simulink model "Rectiafier"  (R2024b)
settings: Solver=VariableStepAuto  StartTime=0.0  StopTime=0.1  RelTol=1e-3
libraries: spsThyristorLib x4, spsVoltageMeasurementLib x3, spsACVoltageSourceLib x1, dspswit3 x1, spsSeriesRLCBranchLib x1, spsUniversalBridgeLib x1, sps_lib x1
settings Model: Creator=Ahmad  LastModifiedBy=Ahmad

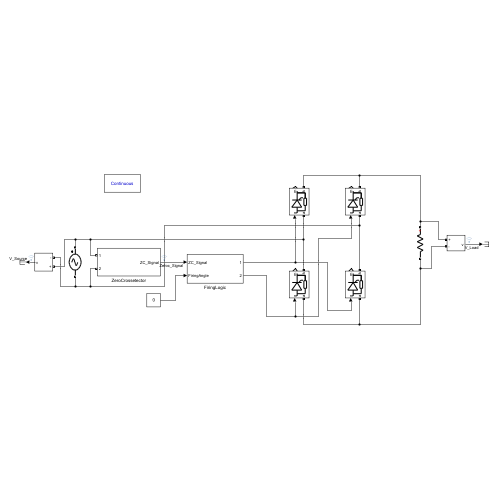
[thumbnail: Simulink's stored preview of the top-level diagram]
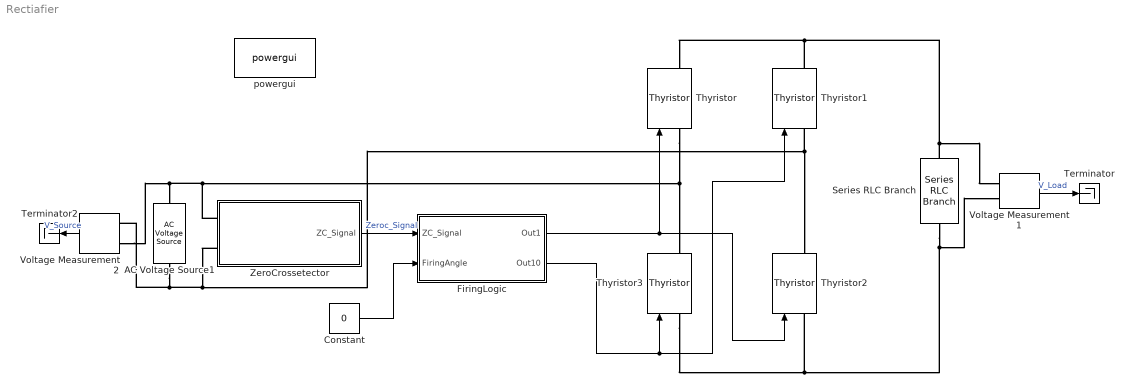
== system Rectiafier ==
  AC Voltage Source1 : spsACVoltageSourceLib/AC Voltage Source  Amplitude=sqrt(2)*220  Phase=0  Frequency=50  SampleTime=0  Measurements=None  BusType=swing  Pref=10e3  Qref=0  Qmin=-inf  Qmax=+inf
  Constant : Constant  Value=0
  FiringLogic : Subsystem
  Series RLC Branch : spsSeriesRLCBranchLib/Series RLC Branch  LConnTagsString=__new0  RConnTagsString=__new0  BranchType=R  Resistance=1  Inductance=1e-3  SetiL0=off  InitialCurrent=0  Capacitance=1e-6  Setx0=off  InitialVoltage=0  Measurements=None
  Terminator : Terminator
  Terminator2 : Terminator
  Thyristor{,1..3} (4 alike) : spsThyristorLib/Thyristor  Ron=0.001  Lon=0  Vf=0.8  IC=0  Rs=500  Cs=250e-9  Measurements=on
  Voltage Measurement1 : spsVoltageMeasurementLib/Voltage Measurement  PhasorSimulation=off  OutputType=Complex  PSBequivalent=0
  Voltage Measurement2 : spsVoltageMeasurementLib/Voltage Measurement  PhasorSimulation=off  OutputType=Complex  PSBequivalent=0
  ZeroCrossetector : Subsystem
  powergui : sps_lib/powergui  Priority=1  SimulationMode=Continuous  SampleTime=50e-6  frequency=60  Iterations=50  frequencyindice=0  Pbase=100e6  ErrMax=1e-4  UnitsV=kV  UnitsW=MW  buscounter=0  FunctionMessages=off  echomessages=off  EnableUseOfTLC=off  CurrentSourceSwitches=off  DisableSnubberDevices=off  DisableRonSwitches=off  DisableVfSwitches=off  DisplayEquations=off  AutomaticDiscreteSolvers=off  SolverType=Tustin/Backward Euler (TBE)  Interpol=off  ExternalGateDelay=off  methode=off  Ts=100  x0status=blocks  SPID=on  SwTol=0  HookPort=off  NonlinearTolerance=1e-4  nMaxIteration=100  ContinueOnMaxIteration=off  RestoreLinks=warning  ResistiveCurrentMeasurement=off  Frange=[0:2:500]  Ylog=off  Xlog=on  ShowGrid=off  save=off  variable=ZData  structure=0  ZoomFFT=off  StartTime=0.0  cycles=1  DisplayStyle=1  fundamental=60  FreqAxis=off  MaxFrequency=1000  frequencyindicesteady=1  RmsSteady=1  display=off
  wires:
  Voltage Measurement1/1 -> Terminator/1  "V_Load"
  Voltage Measurement2/1 -> Terminator2/1  "V_Source"
  ZeroCrossetector/1(ZC_Signal) -> FiringLogic/1(ZC_Signal)  "Zeroc_Signal"
  Constant/1 -> FiringLogic/2(FiringAngle)
  FiringLogic/1(Out1) -> Thyristor2/1, Thyristor/1
  FiringLogic/2(Out10) -> Thyristor1/1, Thyristor3/1
  connections:
  Voltage Measurement2/LConn1 -- ZeroCrossetector/LConn1 -- Thyristor/LConn1 -- Thyristor3/RConn1 -- AC Voltage Source1/RConn1
  AC Voltage Source1/LConn1 -- ZeroCrossetector/LConn2 -- Thyristor1/LConn1 -- Thyristor2/RConn1 -- Voltage Measurement2/LConn2
  Series RLC Branch/RConn1 -- Thyristor3/LConn1 -- Thyristor2/LConn1 -- Voltage Measurement1/LConn2
  Series RLC Branch/LConn1 -- Thyristor1/RConn1 -- Thyristor/RConn1 -- Voltage Measurement1/LConn1

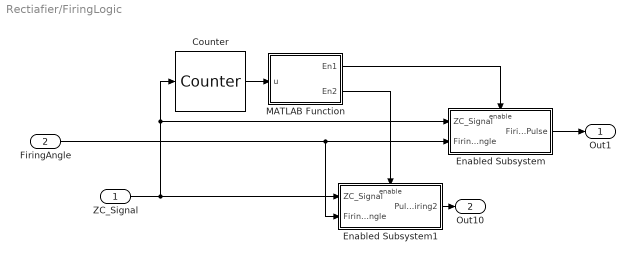
== system Rectiafier/FiringLogic ==
  ZC_Signal : Inport
  FiringAngle : Inport  Port=2
  Counter : dspswit3/Counter  Direction=Up  CountEvent=Rising edge  CounterSize=User defined  MaxCount=255  InitialCount=0  Output=Count  HitValue=32  ResetInput=off  SamplesPerFrame=1  Ts=1  CntDtype=double  HitDtype=Logical
  Enabled Subsystem : Subsystem  TreatAsAtomicUnit=on
  Enabled Subsystem1 : Subsystem  TreatAsAtomicUnit=on
  MATLAB Function : MATLAB Function  TreatAsAtomicUnit=on
  Out1 : Outport
  Out10 : Outport  Port=2
  wires:
  ZC_Signal/1 -> Counter/1, Enabled Subsystem/1(ZC_Signal), Enabled Subsystem1/1(ZC_Signal)
  Counter/1 -> MATLAB Function/1(u)
  MATLAB Function/1(En1) -> Enabled Subsystem/Enable
  MATLAB Function/2(En2) -> Enabled Subsystem1/Enable
  FiringAngle/1 -> Enabled Subsystem1/2(FiringAngle), Enabled Subsystem/2(FiringAngle)
  Enabled Subsystem/1(FiringPulse) -> Out1/1
  Enabled Subsystem1/1(Pulse_Firing2) -> Out10/1

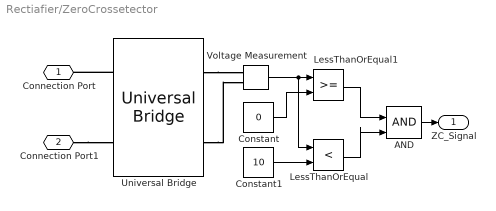
== system Rectiafier/ZeroCrossetector ==
  AND : Logic  IconShape=distinctive  AllPortsSameDT=off  OutDataTypeStr=boolean
  Constant : Constant  Value=0
  Constant1 : Constant  Value=10
  LessThanOrEqual : RelationalOperator  Operator=<  OutDataTypeStr=boolean  RndMeth=Simplest  InputSameDT=off
  LessThanOrEqual1 : RelationalOperator  OutDataTypeStr=boolean  RndMeth=Simplest  InputSameDT=off
  Universal Bridge : spsUniversalBridgeLib/Universal Bridge  Arms=2  SnubberResistance=1e5  SnubberCapacitance=inf  Device=Diodes  Ron=1e-3  Lon=0  ForwardVoltages="[  0  0  ]"  ForwardVoltage=0  GTOparameters=[ 10e-6 , 20e-6 ]  IGBTparameters=[ 1e-6 , 2e-6 ]  Measurements=None  Measurements_2=None  converterType=Rectifier
  Voltage Measurement : spsVoltageMeasurementLib/Voltage Measurement  PhasorSimulation=off  OutputType=Complex  PSBequivalent=0
  Connection Port : PMIOPort  Side=Left
  Connection Port1 : PMIOPort  Port=2  Side=Left
  ZC_Signal : Outport
  wires:
  Voltage Measurement/1 -> LessThanOrEqual/1, LessThanOrEqual1/1
  Constant/1 -> LessThanOrEqual1/2
  Constant1/1 -> LessThanOrEqual/2
  LessThanOrEqual1/1 -> AND/1
  LessThanOrEqual/1 -> AND/2
  AND/1 -> ZC_Signal/1
  connections:
  Universal Bridge/LConn1 -- Connection Port/RConn1
  Connection Port1/RConn1 -- Universal Bridge/LConn2
  Universal Bridge/RConn1 -- Voltage Measurement/LConn1
  Universal Bridge/RConn2 -- Voltage Measurement/LConn2

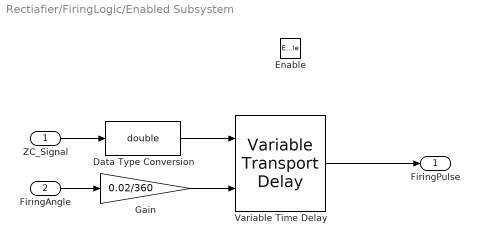
== system Rectiafier/FiringLogic/Enabled Subsystem ==
  ZC_Signal : Inport
  FiringAngle : Inport  Port=2
  Enable : EnablePort
  Data Type Conversion : DataTypeConversion  OutDataTypeStr=double  SaturateOnIntegerOverflow=off  RndMeth=Floor
  Gain : Gain  Gain=0.02/360
  Variable Time Delay : VariableTransportDelay  MaximumDelay=10  MaximumPoints=1400
  FiringPulse : Outport
  wires:
  ZC_Signal/1 -> Data Type Conversion/1
  FiringAngle/1 -> Gain/1
  Gain/1 -> Variable Time Delay/2
  Variable Time Delay/1 -> FiringPulse/1
  Data Type Conversion/1 -> Variable Time Delay/1

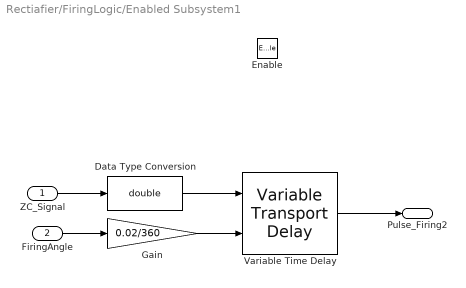
== system Rectiafier/FiringLogic/Enabled Subsystem1 ==
  ZC_Signal : Inport
  FiringAngle : Inport  Port=2
  Enable : EnablePort
  Data Type Conversion : DataTypeConversion  OutDataTypeStr=double  SaturateOnIntegerOverflow=off  RndMeth=Floor
  Gain : Gain  Gain=0.02/360
  Variable Time Delay : VariableTransportDelay  MaximumDelay=10  MaximumPoints=1400
  Pulse_Firing2 : Outport
  wires:
  Gain/1 -> Variable Time Delay/2
  Data Type Conversion/1 -> Variable Time Delay/1
  ZC_Signal/1 -> Data Type Conversion/1
  FiringAngle/1 -> Gain/1
  Variable Time Delay/1 -> Pulse_Firing2/1

== matlab function Rectiafier/FiringLogic/MATLAB Function ==
  data: u input; En1 output; En2 output
function [En1 , En2] = fcn(u)

En1 = 0;
En2 = 0;

if mod(u,2) == 0
   En1 = 1;
   En2 = 0;
end

if mod(u,2) == 1
   En1 = 0;
   En2 = 1;
end
